simulink model "fuzzy_controller_7_trimf"  (Simulink 7.2)
settings: Solver=ode45  StartTime=0.0  StopTime=10.0  RelTol=1e-3
values from neighbouring files (symbols this model uses):
  fi_1_a = -0.786    [fuzzy_controller_3_trimf_params.m]    (also in fuzzy_controller_5_gbell_params.m = 0.1768; fuzzy_controller_5_trimf_optimal_params.m; fuzzy_controller_5_trimf_params.m; fuzzy_controller_7_trimf_params.m)
  fi_1_b = -0.786    [fuzzy_controller_3_trimf_params.m]    (also in fuzzy_controller_5_gbell_params.m = 3.278; fuzzy_controller_5_trimf_optimal_params.m; fuzzy_controller_5_trimf_params.m; fuzzy_controller_7_trimf_params.m)
  fi_1_c = 0    [fuzzy_controller_3_trimf_params.m]    (also in fuzzy_controller_5_gbell_params.m = -0.7664; fuzzy_controller_5_trimf_optimal_params.m = -0.1; fuzzy_controller_5_trimf_params.m = -0.393; fuzzy_controller_7_trimf_params.m = -0.523)
  fi_2_a = -0.786    [fuzzy_controller_3_trimf_params.m]    (also in fuzzy_controller_5_gbell_params.m = 0.1965; fuzzy_controller_5_trimf_optimal_params.m = -0.1; fuzzy_controller_5_trimf_params.m; fuzzy_controller_7_trimf_params.m)
  fi_2_b = 0    [fuzzy_controller_3_trimf_params.m]    (also in fuzzy_controller_5_gbell_params.m = 3.278; fuzzy_controller_5_trimf_optimal_params.m = -0.05; fuzzy_controller_5_trimf_params.m = -0.393; fuzzy_controller_7_trimf_params.m = -0.5238)
  fi_2_c = 0.786    [fuzzy_controller_3_trimf_params.m]    (also in fuzzy_controller_5_gbell_params.m = -0.393; fuzzy_controller_5_trimf_optimal_params.m = 0; fuzzy_controller_5_trimf_params.m = 0; fuzzy_controller_7_trimf_params.m = -0.262)
  fi_3_a = 0    [fuzzy_controller_3_trimf_params.m]    (also in fuzzy_controller_5_gbell_params.m = 0.1965; fuzzy_controller_5_trimf_optimal_params.m = -0.05; fuzzy_controller_5_trimf_params.m = -0.393; fuzzy_controller_7_trimf_params.m = -0.523)
  fi_3_b = 0.786    [fuzzy_controller_3_trimf_params.m]    (also in fuzzy_controller_5_gbell_params.m = 3.278; fuzzy_controller_5_trimf_optimal_params.m = 0; fuzzy_controller_5_trimf_params.m = 0; fuzzy_controller_7_trimf_params.m = -0.262)
  fi_3_c = 0.786    [fuzzy_controller_3_trimf_params.m]    (also in fuzzy_controller_5_gbell_params.m = 0; fuzzy_controller_5_trimf_optimal_params.m = 0.05; fuzzy_controller_5_trimf_params.m = 0.393; fuzzy_controller_7_trimf_params.m = 0)
  fi_4_a = 0.1965    [fuzzy_controller_5_gbell_params.m]    (also in fuzzy_controller_5_trimf_optimal_params.m = 0; fuzzy_controller_5_trimf_params.m = 0; fuzzy_controller_7_trimf_params.m = -0.262)
  fi_4_b = 3.278    [fuzzy_controller_5_gbell_params.m]    (also in fuzzy_controller_5_trimf_optimal_params.m = 0.05; fuzzy_controller_5_trimf_params.m = 0.393; fuzzy_controller_7_trimf_params.m = 0)
  fi_4_c = 0.393    [fuzzy_controller_5_gbell_params.m]    (also in fuzzy_controller_5_trimf_optimal_params.m = 0.1; fuzzy_controller_5_trimf_params.m = 0.786; fuzzy_controller_7_trimf_params.m = 0.262)
  fi_5_a = 0.1768    [fuzzy_controller_5_gbell_params.m]    (also in fuzzy_controller_5_trimf_optimal_params.m = 0.05; fuzzy_controller_5_trimf_params.m = 0.393; fuzzy_controller_7_trimf_params.m = 0)
  fi_5_b = 3.278    [fuzzy_controller_5_gbell_params.m]    (also in fuzzy_controller_5_trimf_optimal_params.m = 0.1; fuzzy_controller_5_trimf_params.m = 0.786; fuzzy_controller_7_trimf_params.m = 0.262)
  fi_5_c = 0.7664    [fuzzy_controller_5_gbell_params.m]    (also in fuzzy_controller_5_trimf_optimal_params.m = 0.786; fuzzy_controller_5_trimf_params.m = 0.786; fuzzy_controller_7_trimf_params.m = 0.523)
  fi_6_a = 0.262    [fuzzy_controller_7_trimf_params.m]
  fi_6_b = 0.523    [fuzzy_controller_7_trimf_params.m]
  fi_6_c = 0.786    [fuzzy_controller_7_trimf_params.m]
  fi_7_a = 0.523    [fuzzy_controller_7_trimf_params.m]
  fi_7_b = 0.786    [fuzzy_controller_7_trimf_params.m]
  fi_7_c = 0.786    [fuzzy_controller_7_trimf_params.m]
  FORCE_1_a = -150    [fuzzy_controller_3_trimf_params.m]    (also in fuzzy_controller_5_trimf_optimal_params.m; fuzzy_controller_5_trimf_params.m; fuzzy_controller_7_trimf_params.m)
  FORCE_1_b = -150    [fuzzy_controller_3_trimf_params.m]    (also in fuzzy_controller_5_trimf_optimal_params.m; fuzzy_controller_5_trimf_params.m; fuzzy_controller_7_trimf_params.m)
  FORCE_1_c = 0    [fuzzy_controller_3_trimf_params.m]    (also in fuzzy_controller_5_trimf_optimal_params.m = -75; fuzzy_controller_5_trimf_params.m = -75; fuzzy_controller_7_trimf_params.m = -100)
  FORCE_2_a = -150    [fuzzy_controller_3_trimf_params.m]    (also in fuzzy_controller_5_trimf_optimal_params.m; fuzzy_controller_5_trimf_params.m; fuzzy_controller_7_trimf_params.m)
  FORCE_2_b = 0    [fuzzy_controller_3_trimf_params.m]    (also in fuzzy_controller_5_trimf_optimal_params.m = -75; fuzzy_controller_5_trimf_params.m = -75; fuzzy_controller_7_trimf_params.m = -100)
  FORCE_2_c = 150    [fuzzy_controller_3_trimf_params.m]    (also in fuzzy_controller_5_trimf_optimal_params.m = 0; fuzzy_controller_5_trimf_params.m = 0; fuzzy_controller_7_trimf_params.m = -50)
  FORCE_3_a = 0    [fuzzy_controller_3_trimf_params.m]    (also in fuzzy_controller_5_trimf_optimal_params.m = -75; fuzzy_controller_5_trimf_params.m = -75; fuzzy_controller_7_trimf_params.m = -100)
  FORCE_3_b = 150    [fuzzy_controller_3_trimf_params.m]    (also in fuzzy_controller_5_trimf_optimal_params.m = 0; fuzzy_controller_5_trimf_params.m = 0; fuzzy_controller_7_trimf_params.m = -50)
  FORCE_3_c = 150    [fuzzy_controller_3_trimf_params.m]    (also in fuzzy_controller_5_trimf_optimal_params.m = 75; fuzzy_controller_5_trimf_params.m = 75; fuzzy_controller_7_trimf_params.m = 0)
  FORCE_4_a = 0    [fuzzy_controller_5_trimf_optimal_params.m]    (also in fuzzy_controller_5_trimf_params.m; fuzzy_controller_7_trimf_params.m = -50)
  FORCE_4_b = 75    [fuzzy_controller_5_trimf_optimal_params.m]    (also in fuzzy_controller_5_trimf_params.m; fuzzy_controller_7_trimf_params.m = 0)
  FORCE_4_c = 150    [fuzzy_controller_5_trimf_optimal_params.m]    (also in fuzzy_controller_5_trimf_params.m; fuzzy_controller_7_trimf_params.m = 50)
  FORCE_5_a = 75    [fuzzy_controller_5_trimf_optimal_params.m]    (also in fuzzy_controller_5_trimf_params.m; fuzzy_controller_7_trimf_params.m = 0)
  FORCE_5_b = 150    [fuzzy_controller_5_trimf_optimal_params.m]    (also in fuzzy_controller_5_trimf_params.m; fuzzy_controller_7_trimf_params.m = 50)
  FORCE_5_c = 150    [fuzzy_controller_5_trimf_optimal_params.m]    (also in fuzzy_controller_5_trimf_params.m; fuzzy_controller_7_trimf_params.m = 100)
  FORCE_6_a = 50    [fuzzy_controller_7_trimf_params.m]
  FORCE_6_b = 100    [fuzzy_controller_7_trimf_params.m]
  FORCE_6_c = 150    [fuzzy_controller_7_trimf_params.m]
  FORCE_7_a = 100    [fuzzy_controller_7_trimf_params.m]
  FORCE_7_b = 150    [fuzzy_controller_7_trimf_params.m]
  FORCE_7_c = 150    [fuzzy_controller_7_trimf_params.m]
  FORCE_Range_1 = -150    [fuzzy_controller_3_trimf_params.m]    (also in fuzzy_controller_5_gauss_params.m; fuzzy_controller_5_gbell_params.m; fuzzy_controller_5_trimf_optimal_params.m; fuzzy_controller_5_trimf_params.m)
  FORCE_Range_2 = 150    [fuzzy_controller_3_trimf_params.m]    (also in fuzzy_controller_5_gauss_params.m; fuzzy_controller_5_gbell_params.m; fuzzy_controller_5_trimf_optimal_params.m; fuzzy_controller_5_trimf_params.m)
  omega_1_a = -1.57    [fuzzy_controller_3_trimf_params.m]    (also in fuzzy_controller_5_gbell_params.m = 0.3532; fuzzy_controller_5_trimf_optimal_params.m; fuzzy_controller_5_trimf_params.m; fuzzy_controller_7_trimf_params.m)
  omega_1_b = -1.57    [fuzzy_controller_3_trimf_params.m]    (also in fuzzy_controller_5_gbell_params.m = 3.278; fuzzy_controller_5_trimf_optimal_params.m; fuzzy_controller_5_trimf_params.m; fuzzy_controller_7_trimf_params.m)
  omega_1_c = 0    [fuzzy_controller_3_trimf_params.m]    (also in fuzzy_controller_5_gbell_params.m = -1.531; fuzzy_controller_5_trimf_optimal_params.m = -0.86; fuzzy_controller_5_trimf_params.m = -0.785; fuzzy_controller_7_trimf_params.m = -1.047)
  omega_2_a = -1.57    [fuzzy_controller_3_trimf_params.m]    (also in fuzzy_controller_5_gbell_params.m = 0.3925; fuzzy_controller_5_trimf_optimal_params.m = -0.86; fuzzy_controller_5_trimf_params.m; fuzzy_controller_7_trimf_params.m)
  omega_2_b = 0    [fuzzy_controller_3_trimf_params.m]    (also in fuzzy_controller_5_gbell_params.m = 3.278; fuzzy_controller_5_trimf_optimal_params.m = -0.43; fuzzy_controller_5_trimf_params.m = -0.785; fuzzy_controller_7_trimf_params.m = -1.047)
  omega_2_c = 1.57    [fuzzy_controller_3_trimf_params.m]    (also in fuzzy_controller_5_gbell_params.m = -0.785; fuzzy_controller_5_trimf_optimal_params.m = 0; fuzzy_controller_5_trimf_params.m = 0; fuzzy_controller_7_trimf_params.m = -0.523)
  omega_3_a = 0    [fuzzy_controller_3_trimf_params.m]    (also in fuzzy_controller_5_gbell_params.m = 0.3925; fuzzy_controller_5_trimf_optimal_params.m = -0.43; fuzzy_controller_5_trimf_params.m = -0.785; fuzzy_controller_7_trimf_params.m = -1.047)
  omega_3_b = 1.57    [fuzzy_controller_3_trimf_params.m]    (also in fuzzy_controller_5_gbell_params.m = 3.278; fuzzy_controller_5_trimf_optimal_params.m = 0; fuzzy_controller_5_trimf_params.m = 0; fuzzy_controller_7_trimf_params.m = -0.523)
  omega_3_c = 1.57    [fuzzy_controller_3_trimf_params.m]    (also in fuzzy_controller_5_gbell_params.m = 0; fuzzy_controller_5_trimf_optimal_params.m = 0.43; fuzzy_controller_5_trimf_params.m = 0.785; fuzzy_controller_7_trimf_params.m = 0)
  omega_4_a = 0.3925    [fuzzy_controller_5_gbell_params.m]    (also in fuzzy_controller_5_trimf_optimal_params.m = 0; fuzzy_controller_5_trimf_params.m = 0; fuzzy_controller_7_trimf_params.m = -0.523)
  omega_4_b = 3.278    [fuzzy_controller_5_gbell_params.m]    (also in fuzzy_controller_5_trimf_optimal_params.m = 0.43; fuzzy_controller_5_trimf_params.m = 0.785; fuzzy_controller_7_trimf_params.m = 0)
  omega_4_c = 0.785    [fuzzy_controller_5_gbell_params.m]    (also in fuzzy_controller_5_trimf_optimal_params.m = 0.86; fuzzy_controller_5_trimf_params.m = 1.57; fuzzy_controller_7_trimf_params.m = 0.523)
  omega_5_a = 0.3532    [fuzzy_controller_5_gbell_params.m]    (also in fuzzy_controller_5_trimf_optimal_params.m = 0.43; fuzzy_controller_5_trimf_params.m = 0.785; fuzzy_controller_7_trimf_params.m = 0)
  omega_5_b = 3.278    [fuzzy_controller_5_gbell_params.m]    (also in fuzzy_controller_5_trimf_optimal_params.m = 0.86; fuzzy_controller_5_trimf_params.m = 1.57; fuzzy_controller_7_trimf_params.m = 0.523)
  omega_5_c = 1.531    [fuzzy_controller_5_gbell_params.m]    (also in fuzzy_controller_5_trimf_optimal_params.m = 1.57; fuzzy_controller_5_trimf_params.m = 1.57; fuzzy_controller_7_trimf_params.m = 1.047)
  omega_6_a = 0.523    [fuzzy_controller_7_trimf_params.m]
  omega_6_b = 1.047    [fuzzy_controller_7_trimf_params.m]
  omega_6_c = 1.57    [fuzzy_controller_7_trimf_params.m]
  omega_7_a = 1.047    [fuzzy_controller_7_trimf_params.m]
  omega_7_b = 1.57    [fuzzy_controller_7_trimf_params.m]
  omega_7_c = 1.57    [fuzzy_controller_7_trimf_params.m]
(part 1 of 4)
settings Model: Creator=Student  ModifiedByFormat=Student  LastModifiedBy=Student
settings OptimizationCC: ExpressionDepthLimit=128
settings DebuggingCC: AlgebraicLoopMsg=error  UnderspecifiedInitializationDetection=Simplified  MergeDetectMultiDrivingBlocksExec=error  SolverPrmCheckMsg=none  FcnCallInpInsideContextMsg=Enable All  StateNameClashWarn=none  StrictBusMsg=ErrorLevel1
settings HardwareCC: ProdBitPerLong=64  ProdIntDivRoundTo=Zero  ProdEndianess=LittleEndian  ProdWordSize=64  ProdHWDeviceType=Intel->x86-64
settings RTWCC: Description=Create Visual C/C++ Solution File for Simulink Coder  GenerateReport=on  RetainRTWFile=on  LaunchReport=on
settings CodeAppCC: ForceParamTrailComments=on  CustomSymbolStrType=$N$R$M_T
settings GRTTargetCC: TargetFunctionLibrary=C99 (ISO)

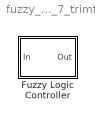
== system fuzzy_controller_7_trimf ==
  Fuzzy Logic Controller : Subsystem

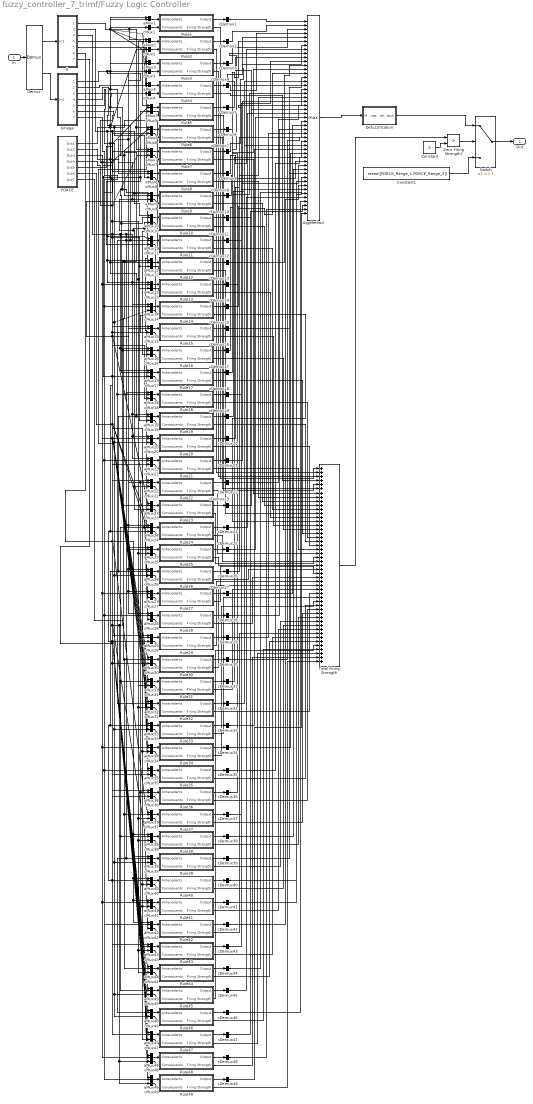
== system fuzzy_controller_7_trimf/Fuzzy Logic Controller ==
  In : Inport
  AggMethod : MinMax  Function=max  Inputs=49  SaturateOnIntegerOverflow=on  InputSameDT=on
  Constant : Constant  Value=0
  Constant1 : Constant  Value=mean([FORCE_Range_1 FORCE_Range_2])
  Defuzzification : Subsystem
  Demux : Demux  Outputs=2
  FORCE : Subsystem
  Rule1 : Subsystem
  Rule10 : Subsystem
  Rule11 : Subsystem
  Rule12 : Subsystem
  Rule13 : Subsystem
  Rule14 : Subsystem
  Rule15 : Subsystem
  Rule16 : Subsystem
  Rule17 : Subsystem
  Rule18 : Subsystem
  Rule19 : Subsystem
  Rule2 : Subsystem
  Rule20 : Subsystem
  Rule21 : Subsystem
  Rule22 : Subsystem
  Rule23 : Subsystem
  Rule24 : Subsystem
  Rule25 : Subsystem
  Rule26 : Subsystem
  Rule27 : Subsystem
  Rule28 : Subsystem
  Rule29 : Subsystem
  Rule3 : Subsystem
  Rule30 : Subsystem
  Rule31 : Subsystem
  Rule32 : Subsystem
  Rule33 : Subsystem
  Rule34 : Subsystem
  Rule35 : Subsystem
  Rule36 : Subsystem
  Rule37 : Subsystem
  Rule38 : Subsystem
  Rule39 : Subsystem
  Rule4 : Subsystem
  Rule40 : Subsystem
  Rule41 : Subsystem
  Rule42 : Subsystem
  Rule43 : Subsystem
  Rule44 : Subsystem
  Rule45 : Subsystem
  Rule46 : Subsystem
  Rule47 : Subsystem
  Rule48 : Subsystem
  Rule49 : Subsystem
  Rule5 : Subsystem
  Rule6 : Subsystem
  Rule7 : Subsystem
  Rule8 : Subsystem
  Rule9 : Subsystem
  Switch : Switch  Threshold=1
  Total Firing Strength : Sum  Inputs=49
  Zero Firing Strength? : RelationalOperator  Operator=>  LogicOutDataTypeMode=boolean  OutDataTypeStr=boolean
  aMux{1..49} (49 alike) : Mux  Inputs=2
  cDemux{1..49} (49 alike) : Demux  Outputs=1
  cMux{1..49} (49 alike) : Mux  Inputs=1
  fi : Subsystem
  omega : Subsystem
  Out : Outport
  wires:
  Total Firing Strength/1 -> Zero Firing Strength?/1
  Constant/1 -> Zero Firing Strength?/2
  Zero Firing Strength?/1 -> Switch/2
  Switch/1 -> Out/1
  Constant1/1 -> Switch/3
  AggMethod/1 -> Defuzzification/1(MF values)
  Defuzzification/1(defuzzified output) -> Switch/1
  Demux/1 -> fi/1(In1)
  In/1 -> Demux/1
  Demux/2 -> omega/1(In1)
  aMux1/1 -> Rule1/1(Antecedents)
  cMux1/1 -> Rule1/2(Consequents)
  fi/1(Out1) -> aMux6/1, aMux7/1, aMux2/1, aMux1/1, aMux3/1, aMux4/1, aMux5/1
  omega/1(Out1) -> aMux36/2, aMux43/2, aMux29/2, aMux22/2, aMux8/2, aMux15/2, aMux1/2
  FORCE/1(Out1) -> cMux15/1, cMux8/1, cMux1/1, cMux2/1
  aMux2/1 -> Rule2/1(Antecedents)
  cMux2/1 -> Rule2/2(Consequents)
  omega/2(Out2) -> aMux16/2, aMux23/2, aMux30/2, aMux37/2, aMux44/2, aMux9/2, aMux2/2
  aMux3/1 -> Rule3/1(Antecedents)
  cMux3/1 -> Rule3/2(Consequents)
  omega/3(Out3) -> aMux10/2, aMux17/2, aMux45/2, aMux38/2, aMux31/2, aMux24/2, aMux3/2
  FORCE/2(Out2) -> cMux22/1, cMux23/1, cMux10/1, cMux16/1, cMux9/1, cMux3/1
  aMux4/1 -> Rule4/1(Antecedents)
  cMux4/1 -> Rule4/2(Consequents)
  omega/4(Out4) -> aMux18/2, aMux25/2, aMux32/2, aMux46/2, aMux39/2, aMux11/2, aMux4/2
  FORCE/3(Out3) -> cMux5/1, cMux11/1, cMux4/1, cMux24/1, cMux30/1, cMux36/1, cMux29/1, cMux17/1
  aMux5/1 -> Rule5/1(Antecedents)
  cMux5/1 -> Rule5/2(Consequents)
  omega/5(Out5) -> aMux5/2, aMux12/2, aMux33/2, aMux47/2, aMux40/2, aMux26/2, aMux19/2
  aMux6/1 -> Rule6/1(Antecedents)
  cMux6/1 -> Rule6/2(Consequents)
  omega/6(Out6) -> aMux48/2, aMux41/2, aMux34/2, aMux27/2, aMux13/2, aMux6/2, aMux20/2
  FORCE/4(Out4) -> cMux19/1, cMux43/1, cMux44/1, cMux38/1, cMux37/1, cMux32/1, cMux25/1, cMux31/1, cMux18/1, cMux12/1, cMux13/1, cMux6/1, cMux7/1
  aMux7/1 -> Rule7/1(Antecedents)
  cMux7/1 -> Rule7/2(Consequents)
  omega/7(Out7) -> aMux49/2, aMux35/2, aMux28/2, aMux21/2, aMux14/2, aMux7/2, aMux42/2
  aMux8/1 -> Rule8/1(Antecedents)
  cMux8/1 -> Rule8/2(Consequents)
  fi/2(Out2) -> aMux9/1, aMux10/1, aMux8/1, aMux13/1, aMux14/1, aMux12/1, aMux11/1
  aMux9/1 -> Rule9/1(Antecedents)
  cMux9/1 -> Rule9/2(Consequents)
  aMux10/1 -> Rule10/1(Antecedents)
  cMux10/1 -> Rule10/2(Consequents)
  aMux11/1 -> Rule11/1(Antecedents)
  cMux11/1 -> Rule11/2(Consequents)
  aMux12/1 -> Rule12/1(Antecedents)
  cMux12/1 -> Rule12/2(Consequents)
  aMux13/1 -> Rule13/1(Antecedents)
  cMux13/1 -> Rule13/2(Consequents)
  aMux14/1 -> Rule14/1(Antecedents)
  cMux14/1 -> Rule14/2(Consequents)
  FORCE/5(Out5) -> cMux26/1, cMux45/1, cMux46/1, cMux39/1, cMux33/1, cMux20/1, cMux14/1
  aMux15/1 -> Rule15/1(Antecedents)
  cMux15/1 -> Rule15/2(Consequents)
  fi/3(Out3) -> aMux21/1, aMux20/1, aMux19/1, aMux18/1, aMux16/1, aMux17/1, aMux15/1
  aMux16/1 -> Rule16/1(Antecedents)
  cMux16/1 -> Rule16/2(Consequents)
  aMux17/1 -> Rule17/1(Antecedents)
  cMux17/1 -> Rule17/2(Consequents)
  aMux18/1 -> Rule18/1(Antecedents)
  cMux18/1 -> Rule18/2(Consequents)
  aMux19/1 -> Rule19/1(Antecedents)
  cMux19/1 -> Rule19/2(Consequents)
  aMux20/1 -> Rule20/1(Antecedents)
  cMux20/1 -> Rule20/2(Consequents)
  aMux21/1 -> Rule21/1(Antecedents)
  cMux21/1 -> Rule21/2(Consequents)
  FORCE/6(Out6) -> cMux41/1, cMux47/1, cMux40/1, cMux34/1, cMux21/1, cMux27/1, cMux28/1
  aMux22/1 -> Rule22/1(Antecedents)
  cMux22/1 -> Rule22/2(Consequents)
  fi/4(Out4) -> aMux27/1, aMux28/1, aMux26/1, aMux25/1, aMux24/1, aMux22/1, aMux23/1
  aMux23/1 -> Rule23/1(Antecedents)
  cMux23/1 -> Rule23/2(Consequents)
  aMux24/1 -> Rule24/1(Antecedents)
  cMux24/1 -> Rule24/2(Consequents)
  aMux25/1 -> Rule25/1(Antecedents)
  cMux25/1 -> Rule25/2(Consequents)
  aMux26/1 -> Rule26/1(Antecedents)
  cMux26/1 -> Rule26/2(Consequents)
  aMux27/1 -> Rule27/1(Antecedents)
  cMux27/1 -> Rule27/2(Consequents)
  aMux28/1 -> Rule28/1(Antecedents)
  cMux28/1 -> Rule28/2(Consequents)
  aMux29/1 -> Rule29/1(Antecedents)
  cMux29/1 -> Rule29/2(Consequents)
  fi/5(Out5) -> aMux29/1, aMux30/1, aMux31/1, aMux32/1, aMux33/1, aMux34/1, aMux35/1
  aMux30/1 -> Rule30/1(Antecedents)
  cMux30/1 -> Rule30/2(Consequents)
  aMux31/1 -> Rule31/1(Antecedents)
  cMux31/1 -> Rule31/2(Consequents)
  aMux32/1 -> Rule32/1(Antecedents)
  cMux32/1 -> Rule32/2(Consequents)
  aMux33/1 -> Rule33/1(Antecedents)
  cMux33/1 -> Rule33/2(Consequents)
  aMux34/1 -> Rule34/1(Antecedents)
  cMux34/1 -> Rule34/2(Consequents)
  aMux35/1 -> Rule35/1(Antecedents)
  cMux35/1 -> Rule35/2(Consequents)
  FORCE/7(Out7) -> cMux48/1, cMux49/1, cMux35/1, cMux42/1
  aMux36/1 -> Rule36/1(Antecedents)
  cMux36/1 -> Rule36/2(Consequents)
  fi/6(Out6) -> aMux38/1, aMux39/1, aMux40/1, aMux41/1, aMux42/1, aMux36/1, aMux37/1
  aMux37/1 -> Rule37/1(Antecedents)
  cMux37/1 -> Rule37/2(Consequents)
  aMux38/1 -> Rule38/1(Antecedents)
  cMux38/1 -> Rule38/2(Consequents)
  aMux39/1 -> Rule39/1(Antecedents)
  cMux39/1 -> Rule39/2(Consequents)
  aMux40/1 -> Rule40/1(Antecedents)
  cMux40/1 -> Rule40/2(Consequents)
  aMux41/1 -> Rule41/1(Antecedents)
  cMux41/1 -> Rule41/2(Consequents)
  aMux42/1 -> Rule42/1(Antecedents)
  cMux42/1 -> Rule42/2(Consequents)
  aMux43/1 -> Rule43/1(Antecedents)
  cMux43/1 -> Rule43/2(Consequents)
  fi/7(Out7) -> aMux43/1, aMux44/1, aMux45/1, aMux46/1, aMux47/1, aMux48/1, aMux49/1
  aMux44/1 -> Rule44/1(Antecedents)
  cMux44/1 -> Rule44/2(Consequents)
  aMux45/1 -> Rule45/1(Antecedents)
  cMux45/1 -> Rule45/2(Consequents)
  aMux46/1 -> Rule46/1(Antecedents)
  cMux46/1 -> Rule46/2(Consequents)
  aMux47/1 -> Rule47/1(Antecedents)
  cMux47/1 -> Rule47/2(Consequents)
  aMux48/1 -> Rule48/1(Antecedents)
  cMux48/1 -> Rule48/2(Consequents)
  aMux49/1 -> Rule49/1(Antecedents)
  cMux49/1 -> Rule49/2(Consequents)
  cDemux1/1 -> AggMethod/1
  cDemux2/1 -> AggMethod/2
  cDemux3/1 -> AggMethod/3
  cDemux4/1 -> AggMethod/4
  cDemux5/1 -> AggMethod/5
  cDemux6/1 -> AggMethod/6
  cDemux7/1 -> AggMethod/7
  cDemux8/1 -> AggMethod/8
  cDemux9/1 -> AggMethod/9
  cDemux10/1 -> AggMethod/10
  cDemux11/1 -> AggMethod/11
  cDemux12/1 -> AggMethod/12
  cDemux13/1 -> AggMethod/13
  cDemux14/1 -> AggMethod/14
  cDemux15/1 -> AggMethod/15
  cDemux16/1 -> AggMethod/16
  cDemux17/1 -> AggMethod/17
  cDemux18/1 -> AggMethod/18
  cDemux19/1 -> AggMethod/19
  cDemux20/1 -> AggMethod/20
  cDemux21/1 -> AggMethod/21
  cDemux22/1 -> AggMethod/22
  cDemux23/1 -> AggMethod/23
  cDemux24/1 -> AggMethod/24
  cDemux25/1 -> AggMethod/25
  cDemux26/1 -> AggMethod/26
  cDemux27/1 -> AggMethod/27
  cDemux28/1 -> AggMethod/28
  cDemux29/1 -> AggMethod/29
  cDemux30/1 -> AggMethod/30
  cDemux31/1 -> AggMethod/31
  cDemux32/1 -> AggMethod/32
  cDemux33/1 -> AggMethod/33
  cDemux34/1 -> AggMethod/34
  cDemux35/1 -> AggMethod/35
  cDemux36/1 -> AggMethod/36
  cDemux37/1 -> AggMethod/37
  cDemux38/1 -> AggMethod/38
  cDemux39/1 -> AggMethod/39
  cDemux40/1 -> AggMethod/40
  cDemux41/1 -> AggMethod/41
  cDemux42/1 -> AggMethod/42
  cDemux43/1 -> AggMethod/43
  cDemux44/1 -> AggMethod/44
  cDemux45/1 -> AggMethod/45
  cDemux46/1 -> AggMethod/46
  cDemux47/1 -> AggMethod/47
  cDemux48/1 -> AggMethod/48
  cDemux49/1 -> AggMethod/49
  Rule1/1(Output) -> cDemux1/1
  Rule2/1(Output) -> cDemux2/1
  Rule3/1(Output) -> cDemux3/1
  Rule4/1(Output) -> cDemux4/1
  Rule5/1(Output) -> cDemux5/1
  Rule6/1(Output) -> cDemux6/1
  Rule49/1(Output) -> cDemux49/1
  Rule48/1(Output) -> cDemux48/1
  Rule47/1(Output) -> cDemux47/1
  Rule46/1(Output) -> cDemux46/1
  Rule45/1(Output) -> cDemux45/1
  Rule44/1(Output) -> cDemux44/1
  Rule42/1(Output) -> cDemux42/1
  Rule41/1(Output) -> cDemux41/1
  Rule43/1(Output) -> cDemux43/1
  Rule40/1(Output) -> cDemux40/1
  Rule39/1(Output) -> cDemux39/1
  Rule38/1(Output) -> cDemux38/1
  Rule36/1(Output) -> cDemux36/1
  Rule37/1(Output) -> cDemux37/1
  Rule35/1(Output) -> cDemux35/1
  Rule34/1(Output) -> cDemux34/1
  Rule33/1(Output) -> cDemux33/1
  Rule31/1(Output) -> cDemux31/1
  Rule32/1(Output) -> cDemux32/1
  Rule30/1(Output) -> cDemux30/1
  Rule29/1(Output) -> cDemux29/1
  Rule28/1(Output) -> cDemux28/1
  Rule27/1(Output) -> cDemux27/1
  Rule26/1(Output) -> cDemux26/1
  Rule25/1(Output) -> cDemux25/1
  Rule24/1(Output) -> cDemux24/1
  Rule23/1(Output) -> cDemux23/1
  Rule22/1(Output) -> cDemux22/1
  Rule21/1(Output) -> cDemux21/1
  Rule20/1(Output) -> cDemux20/1
  Rule19/1(Output) -> cDemux19/1
  Rule18/1(Output) -> cDemux18/1
  Rule17/1(Output) -> cDemux17/1
  Rule16/1(Output) -> cDemux16/1
  Rule15/1(Output) -> cDemux15/1
  Rule14/1(Output) -> cDemux14/1
  Rule13/1(Output) -> cDemux13/1
  Rule7/1(Output) -> cDemux7/1
  Rule8/1(Output) -> cDemux8/1
  Rule9/1(Output) -> cDemux9/1
  Rule10/1(Output) -> cDemux10/1
  Rule11/1(Output) -> cDemux11/1
  Rule12/1(Output) -> cDemux12/1
  Rule1/2(Firing Strength) -> Total Firing Strength/1
  Rule2/2(Firing Strength) -> Total Firing Strength/2
  Rule3/2(Firing Strength) -> Total Firing Strength/3
  Rule4/2(Firing Strength) -> Total Firing Strength/4
  Rule5/2(Firing Strength) -> Total Firing Strength/5
  Rule6/2(Firing Strength) -> Total Firing Strength/6
  Rule7/2(Firing Strength) -> Total Firing Strength/7
  Rule8/2(Firing Strength) -> Total Firing Strength/8
  Rule9/2(Firing Strength) -> Total Firing Strength/9
  Rule10/2(Firing Strength) -> Total Firing Strength/10
  Rule11/2(Firing Strength) -> Total Firing Strength/11
  Rule12/2(Firing Strength) -> Total Firing Strength/12
  Rule13/2(Firing Strength) -> Total Firing Strength/13
  Rule14/2(Firing Strength) -> Total Firing Strength/14
  Rule15/2(Firing Strength) -> Total Firing Strength/15
  Rule16/2(Firing Strength) -> Total Firing Strength/16
  Rule17/2(Firing Strength) -> Total Firing Strength/17
  Rule18/2(Firing Strength) -> Total Firing Strength/18
  Rule19/2(Firing Strength) -> Total Firing Strength/19
  Rule20/2(Firing Strength) -> Total Firing Strength/20
  Rule21/2(Firing Strength) -> Total Firing Strength/21
  Rule22/2(Firing Strength) -> Total Firing Strength/22
  Rule23/2(Firing Strength) -> Total Firing Strength/23
  Rule24/2(Firing Strength) -> Total Firing Strength/24
  Rule25/2(Firing Strength) -> Total Firing Strength/25
  Rule26/2(Firing Strength) -> Total Firing Strength/26
  Rule27/2(Firing Strength) -> Total Firing Strength/27
  Rule28/2(Firing Strength) -> Total Firing Strength/28
  Rule29/2(Firing Strength) -> Total Firing Strength/29
  Rule30/2(Firing Strength) -> Total Firing Strength/30
  Rule31/2(Firing Strength) -> Total Firing Strength/31
  Rule32/2(Firing Strength) -> Total Firing Strength/32
  Rule33/2(Firing Strength) -> Total Firing Strength/33
  Rule34/2(Firing Strength) -> Total Firing Strength/34
  Rule35/2(Firing Strength) -> Total Firing Strength/35
  Rule36/2(Firing Strength) -> Total Firing Strength/36
  Rule37/2(Firing Strength) -> Total Firing Strength/37
  Rule38/2(Firing Strength) -> Total Firing Strength/38
  Rule39/2(Firing Strength) -> Total Firing Strength/39
  Rule40/2(Firing Strength) -> Total Firing Strength/40
  Rule41/2(Firing Strength) -> Total Firing Strength/41
  Rule42/2(Firing Strength) -> Total Firing Strength/42
  Rule43/2(Firing Strength) -> Total Firing Strength/43
  Rule44/2(Firing Strength) -> Total Firing Strength/44
  Rule45/2(Firing Strength) -> Total Firing Strength/45
  Rule46/2(Firing Strength) -> Total Firing Strength/46
  Rule47/2(Firing Strength) -> Total Firing Strength/47
  Rule48/2(Firing Strength) -> Total Firing Strength/48
  Rule49/2(Firing Strength) -> Total Firing Strength/49

== system fuzzy_controller_7_trimf/Fuzzy Logic Controller/Defuzzification ==
  MF values : Inport
  Action: One : Subsystem  TreatAsAtomicUnit=on
  Action: u1 : Subsystem  TreatAsAtomicUnit=on
  Averaging (COA) : Product  Inputs=*/  SaturateOnIntegerOverflow=on  RndMeth=Zero  InputSameDT=on  OutDataTypeStr=Inherit: Same as first input
  Constant1 : Constant  Value=linspace(FORCE_Range_1,FORCE_Range_2,200)
  If : If  IfExpression=u1 <= 0
  Merge : Merge  InitialOutput=0
  Product (COA) : Product  SaturateOnIntegerOverflow=on  RndMeth=Zero  InputSameDT=on  OutDataTypeStr=Inherit: Same as first input
  Sum : Sum  Inputs=+  SaturateOnIntegerOverflow=on  InputSameDT=on  OutDataTypeStr=Inherit: Same as first input
  Sum1 : Sum  Inputs=+  SaturateOnIntegerOverflow=on  InputSameDT=on  OutDataTypeStr=Inherit: Same as first input
  defuzzified output : Outport
  wires:
  Merge/1 -> Averaging (COA)/2
  Action: u1/1(u2) -> Merge/2
  Action: One/1(Out1) -> Merge/1
  If/1 -> Action: One/Action
  If/2 -> Action: u1/Action
  Sum1/1 -> Action: u1/1(u1), If/1
  Constant1/1 -> Product (COA)/1
  Product (COA)/1 -> Sum/1
  MF values/1 -> Product (COA)/2, Sum1/1
  Sum/1 -> Averaging (COA)/1
  Averaging (COA)/1 -> defuzzified output/1

== system fuzzy_controller_7_trimf/Fuzzy Logic Controller/FORCE ==
  Constant2 : Constant  Value=linspace(FORCE_Range_1,FORCE_Range_2,200)
  tri mf1 : Subsystem  mask{a=FORCE_1_a, b=FORCE_1_b, c=FORCE_1_c}
      mask prompts: a "Left base point a:"; b "Peak location b:"; c "Right base point c:"
  tri mf2 : Subsystem  mask{a=FORCE_2_a, b=FORCE_2_b, c=FORCE_2_c}
      mask prompts: a "Left base point a:"; b "Peak location b:"; c "Right base point c:"
  tri mf3 : Subsystem  mask{a=FORCE_3_a, b=FORCE_3_b, c=FORCE_3_c}
      mask prompts: a "Left base point a:"; b "Peak location b:"; c "Right base point c:"
  tri mf4 : Subsystem  mask{a=FORCE_4_a, b=FORCE_4_b, c=FORCE_4_c}
      mask prompts: a "Left base point a:"; b "Peak location b:"; c "Right base point c:"
  tri mf5 : Subsystem  mask{a=FORCE_5_a, b=FORCE_5_b, c=FORCE_5_c}
      mask prompts: a "Left base point a:"; b "Peak location b:"; c "Right base point c:"
  tri mf6 : Subsystem  mask{a=FORCE_6_a, b=FORCE_6_b, c=FORCE_6_c}
      mask prompts: a "Left base point a:"; b "Peak location b:"; c "Right base point c:"
  tri mf7 : Subsystem  mask{a=FORCE_7_a, b=FORCE_7_b, c=FORCE_7_c}
      mask prompts: a "Left base point a:"; b "Peak location b:"; c "Right base point c:"
  Out1 : Outport
  Out2 : Outport  Port=2
  Out3 : Outport  Port=3
  Out4 : Outport  Port=4
  Out5 : Outport  Port=5
  Out6 : Outport  Port=6
  Out7 : Outport  Port=7
  wires:
  Constant2/1 -> tri mf4/1(x), tri mf6/1(x), tri mf7/1(x), tri mf5/1(x), tri mf3/1(x), tri mf1/1(x), tri mf2/1(x)
  tri mf1/1(MF) -> Out1/1
  tri mf2/1(MF) -> Out2/1
  tri mf3/1(MF) -> Out3/1
  tri mf4/1(MF) -> Out4/1
  tri mf5/1(MF) -> Out5/1
  tri mf6/1(MF) -> Out6/1
  tri mf7/1(MF) -> Out7/1

== system fuzzy_controller_7_trimf/Fuzzy Logic Controller/Rule1 ==
  Antecedents : Inport
  Consequents : Inport  Port=2
  Weight : Constant
  Weighting : Product  SaturateOnIntegerOverflow=on  RndMeth=Zero  InputSameDT=on  OutDataTypeStr=Inherit: Same as first input
  andorMethod : MinMax  SaturateOnIntegerOverflow=on  InputSameDT=on
  impMethod : MinMax  Inputs=2  SaturateOnIntegerOverflow=on  InputSameDT=on
  Output : Outport
  Firing Strength : Outport  Port=2
  wires:
  impMethod/1 -> Output/1
  Weighting/1 -> Firing Strength/1, impMethod/1
  Consequents/1 -> impMethod/2
  Weight/1 -> Weighting/1
  andorMethod/1 -> Weighting/2
  Antecedents/1 -> andorMethod/1

== system fuzzy_controller_7_trimf/Fuzzy Logic Controller/Rule10 ==
  Antecedents : Inport
  Consequents : Inport  Port=2
  Weight : Constant
  Weighting : Product  SaturateOnIntegerOverflow=on  RndMeth=Zero  InputSameDT=on  OutDataTypeStr=Inherit: Same as first input
  andorMethod : MinMax  SaturateOnIntegerOverflow=on  InputSameDT=on
  impMethod : MinMax  Inputs=2  SaturateOnIntegerOverflow=on  InputSameDT=on
  Output : Outport
  Firing Strength : Outport  Port=2
  wires:
  impMethod/1 -> Output/1
  Weighting/1 -> Firing Strength/1, impMethod/1
  Consequents/1 -> impMethod/2
  Weight/1 -> Weighting/1
  andorMethod/1 -> Weighting/2
  Antecedents/1 -> andorMethod/1

== system fuzzy_controller_7_trimf/Fuzzy Logic Controller/Rule11 ==
  Antecedents : Inport
  Consequents : Inport  Port=2
  Weight : Constant
  Weighting : Product  SaturateOnIntegerOverflow=on  RndMeth=Zero  InputSameDT=on  OutDataTypeStr=Inherit: Same as first input
  andorMethod : MinMax  SaturateOnIntegerOverflow=on  InputSameDT=on
  impMethod : MinMax  Inputs=2  SaturateOnIntegerOverflow=on  InputSameDT=on
  Output : Outport
  Firing Strength : Outport  Port=2
  wires:
  impMethod/1 -> Output/1
  Weighting/1 -> Firing Strength/1, impMethod/1
  Consequents/1 -> impMethod/2
  Weight/1 -> Weighting/1
  andorMethod/1 -> Weighting/2
  Antecedents/1 -> andorMethod/1

== system fuzzy_controller_7_trimf/Fuzzy Logic Controller/Rule12 ==
  Antecedents : Inport
  Consequents : Inport  Port=2
  Weight : Constant
  Weighting : Product  SaturateOnIntegerOverflow=on  RndMeth=Zero  InputSameDT=on  OutDataTypeStr=Inherit: Same as first input
  andorMethod : MinMax  SaturateOnIntegerOverflow=on  InputSameDT=on
  impMethod : MinMax  Inputs=2  SaturateOnIntegerOverflow=on  InputSameDT=on
  Output : Outport
  Firing Strength : Outport  Port=2
  wires:
  impMethod/1 -> Output/1
  Weighting/1 -> Firing Strength/1, impMethod/1
  Consequents/1 -> impMethod/2
  Weight/1 -> Weighting/1
  andorMethod/1 -> Weighting/2
  Antecedents/1 -> andorMethod/1

== system fuzzy_controller_7_trimf/Fuzzy Logic Controller/Rule13 ==
  Antecedents : Inport
  Consequents : Inport  Port=2
  Weight : Constant
  Weighting : Product  SaturateOnIntegerOverflow=on  RndMeth=Zero  InputSameDT=on  OutDataTypeStr=Inherit: Same as first input
  andorMethod : MinMax  SaturateOnIntegerOverflow=on  InputSameDT=on
  impMethod : MinMax  Inputs=2  SaturateOnIntegerOverflow=on  InputSameDT=on
  Output : Outport
  Firing Strength : Outport  Port=2
  wires:
  impMethod/1 -> Output/1
  Weighting/1 -> Firing Strength/1, impMethod/1
  Consequents/1 -> impMethod/2
  Weight/1 -> Weighting/1
  andorMethod/1 -> Weighting/2
  Antecedents/1 -> andorMethod/1

== system fuzzy_controller_7_trimf/Fuzzy Logic Controller/Rule14 ==
  Antecedents : Inport
  Consequents : Inport  Port=2
  Weight : Constant
  Weighting : Product  SaturateOnIntegerOverflow=on  RndMeth=Zero  InputSameDT=on  OutDataTypeStr=Inherit: Same as first input
  andorMethod : MinMax  SaturateOnIntegerOverflow=on  InputSameDT=on
  impMethod : MinMax  Inputs=2  SaturateOnIntegerOverflow=on  InputSameDT=on
  Output : Outport
  Firing Strength : Outport  Port=2
  wires:
  impMethod/1 -> Output/1
  Weighting/1 -> Firing Strength/1, impMethod/1
  Consequents/1 -> impMethod/2
  Weight/1 -> Weighting/1
  andorMethod/1 -> Weighting/2
  Antecedents/1 -> andorMethod/1

== system fuzzy_controller_7_trimf/Fuzzy Logic Controller/Rule15 ==
  Antecedents : Inport
  Consequents : Inport  Port=2
  Weight : Constant
  Weighting : Product  SaturateOnIntegerOverflow=on  RndMeth=Zero  InputSameDT=on  OutDataTypeStr=Inherit: Same as first input
  andorMethod : MinMax  SaturateOnIntegerOverflow=on  InputSameDT=on
  impMethod : MinMax  Inputs=2  SaturateOnIntegerOverflow=on  InputSameDT=on
  Output : Outport
  Firing Strength : Outport  Port=2
  wires:
  impMethod/1 -> Output/1
  Weighting/1 -> Firing Strength/1, impMethod/1
  Consequents/1 -> impMethod/2
  Weight/1 -> Weighting/1
  andorMethod/1 -> Weighting/2
  Antecedents/1 -> andorMethod/1

== system fuzzy_controller_7_trimf/Fuzzy Logic Controller/Rule16 ==
  Antecedents : Inport
  Consequents : Inport  Port=2
  Weight : Constant
  Weighting : Product  SaturateOnIntegerOverflow=on  RndMeth=Zero  InputSameDT=on  OutDataTypeStr=Inherit: Same as first input
  andorMethod : MinMax  SaturateOnIntegerOverflow=on  InputSameDT=on
  impMethod : MinMax  Inputs=2  SaturateOnIntegerOverflow=on  InputSameDT=on
  Output : Outport
  Firing Strength : Outport  Port=2
  wires:
  impMethod/1 -> Output/1
  Weighting/1 -> Firing Strength/1, impMethod/1
  Consequents/1 -> impMethod/2
  Weight/1 -> Weighting/1
  andorMethod/1 -> Weighting/2
  Antecedents/1 -> andorMethod/1

== system fuzzy_controller_7_trimf/Fuzzy Logic Controller/Rule17 ==
  Antecedents : Inport
  Consequents : Inport  Port=2
  Weight : Constant
  Weighting : Product  SaturateOnIntegerOverflow=on  RndMeth=Zero  InputSameDT=on  OutDataTypeStr=Inherit: Same as first input
  andorMethod : MinMax  SaturateOnIntegerOverflow=on  InputSameDT=on
  impMethod : MinMax  Inputs=2  SaturateOnIntegerOverflow=on  InputSameDT=on
  Output : Outport
  Firing Strength : Outport  Port=2
  wires:
  impMethod/1 -> Output/1
  Weighting/1 -> Firing Strength/1, impMethod/1
  Consequents/1 -> impMethod/2
  Weight/1 -> Weighting/1
  andorMethod/1 -> Weighting/2
  Antecedents/1 -> andorMethod/1

== system fuzzy_controller_7_trimf/Fuzzy Logic Controller/Rule18 ==
  Antecedents : Inport
  Consequents : Inport  Port=2
  Weight : Constant
  Weighting : Product  SaturateOnIntegerOverflow=on  RndMeth=Zero  InputSameDT=on  OutDataTypeStr=Inherit: Same as first input
  andorMethod : MinMax  SaturateOnIntegerOverflow=on  InputSameDT=on
  impMethod : MinMax  Inputs=2  SaturateOnIntegerOverflow=on  InputSameDT=on
  Output : Outport
  Firing Strength : Outport  Port=2
  wires:
  impMethod/1 -> Output/1
  Weighting/1 -> Firing Strength/1, impMethod/1
  Consequents/1 -> impMethod/2
  Weight/1 -> Weighting/1
  andorMethod/1 -> Weighting/2
  Antecedents/1 -> andorMethod/1

== system fuzzy_controller_7_trimf/Fuzzy Logic Controller/Rule19 ==
  Antecedents : Inport
  Consequents : Inport  Port=2
  Weight : Constant
  Weighting : Product  SaturateOnIntegerOverflow=on  RndMeth=Zero  InputSameDT=on  OutDataTypeStr=Inherit: Same as first input
  andorMethod : MinMax  SaturateOnIntegerOverflow=on  InputSameDT=on
  impMethod : MinMax  Inputs=2  SaturateOnIntegerOverflow=on  InputSameDT=on
  Output : Outport
  Firing Strength : Outport  Port=2
  wires:
  impMethod/1 -> Output/1
  Weighting/1 -> Firing Strength/1, impMethod/1
  Consequents/1 -> impMethod/2
  Weight/1 -> Weighting/1
  andorMethod/1 -> Weighting/2
  Antecedents/1 -> andorMethod/1

== system fuzzy_controller_7_trimf/Fuzzy Logic Controller/Rule2 ==
  Antecedents : Inport
  Consequents : Inport  Port=2
  Weight : Constant
  Weighting : Product  SaturateOnIntegerOverflow=on  RndMeth=Zero  InputSameDT=on  OutDataTypeStr=Inherit: Same as first input
  andorMethod : MinMax  SaturateOnIntegerOverflow=on  InputSameDT=on
  impMethod : MinMax  Inputs=2  SaturateOnIntegerOverflow=on  InputSameDT=on
  Output : Outport
  Firing Strength : Outport  Port=2
  wires:
  impMethod/1 -> Output/1
  Weighting/1 -> Firing Strength/1, impMethod/1
  Consequents/1 -> impMethod/2
  Weight/1 -> Weighting/1
  andorMethod/1 -> Weighting/2
  Antecedents/1 -> andorMethod/1

== system fuzzy_controller_7_trimf/Fuzzy Logic Controller/Rule20 ==
  Antecedents : Inport
  Consequents : Inport  Port=2
  Weight : Constant
  Weighting : Product  SaturateOnIntegerOverflow=on  RndMeth=Zero  InputSameDT=on  OutDataTypeStr=Inherit: Same as first input
  andorMethod : MinMax  SaturateOnIntegerOverflow=on  InputSameDT=on
  impMethod : MinMax  Inputs=2  SaturateOnIntegerOverflow=on  InputSameDT=on
  Output : Outport
  Firing Strength : Outport  Port=2
  wires:
  impMethod/1 -> Output/1
  Weighting/1 -> Firing Strength/1, impMethod/1
  Consequents/1 -> impMethod/2
  Weight/1 -> Weighting/1
  andorMethod/1 -> Weighting/2
  Antecedents/1 -> andorMethod/1

== system fuzzy_controller_7_trimf/Fuzzy Logic Controller/Rule21 ==
  Antecedents : Inport
  Consequents : Inport  Port=2
  Weight : Constant
  Weighting : Product  SaturateOnIntegerOverflow=on  RndMeth=Zero  InputSameDT=on  OutDataTypeStr=Inherit: Same as first input
  andorMethod : MinMax  SaturateOnIntegerOverflow=on  InputSameDT=on
  impMethod : MinMax  Inputs=2  SaturateOnIntegerOverflow=on  InputSameDT=on
  Output : Outport
  Firing Strength : Outport  Port=2
  wires:
  impMethod/1 -> Output/1
  Weighting/1 -> Firing Strength/1, impMethod/1
  Consequents/1 -> impMethod/2
  Weight/1 -> Weighting/1
  andorMethod/1 -> Weighting/2
  Antecedents/1 -> andorMethod/1

== system fuzzy_controller_7_trimf/Fuzzy Logic Controller/Rule22 ==
  Antecedents : Inport
  Consequents : Inport  Port=2
  Weight : Constant
  Weighting : Product  SaturateOnIntegerOverflow=on  RndMeth=Zero  InputSameDT=on  OutDataTypeStr=Inherit: Same as first input
  andorMethod : MinMax  SaturateOnIntegerOverflow=on  InputSameDT=on
  impMethod : MinMax  Inputs=2  SaturateOnIntegerOverflow=on  InputSameDT=on
  Output : Outport
  Firing Strength : Outport  Port=2
  wires:
  impMethod/1 -> Output/1
  Weighting/1 -> Firing Strength/1, impMethod/1
  Consequents/1 -> impMethod/2
  Weight/1 -> Weighting/1
  andorMethod/1 -> Weighting/2
  Antecedents/1 -> andorMethod/1

== system fuzzy_controller_7_trimf/Fuzzy Logic Controller/Rule23 ==
  Antecedents : Inport
  Consequents : Inport  Port=2
  Weight : Constant
  Weighting : Product  SaturateOnIntegerOverflow=on  RndMeth=Zero  InputSameDT=on  OutDataTypeStr=Inherit: Same as first input
  andorMethod : MinMax  SaturateOnIntegerOverflow=on  InputSameDT=on
  impMethod : MinMax  Inputs=2  SaturateOnIntegerOverflow=on  InputSameDT=on
  Output : Outport
  Firing Strength : Outport  Port=2
  wires:
  impMethod/1 -> Output/1
  Weighting/1 -> Firing Strength/1, impMethod/1
  Consequents/1 -> impMethod/2
  Weight/1 -> Weighting/1
  andorMethod/1 -> Weighting/2
  Antecedents/1 -> andorMethod/1

== system fuzzy_controller_7_trimf/Fuzzy Logic Controller/Rule24 ==
  Antecedents : Inport
  Consequents : Inport  Port=2
  Weight : Constant
  Weighting : Product  SaturateOnIntegerOverflow=on  RndMeth=Zero  InputSameDT=on  OutDataTypeStr=Inherit: Same as first input
  andorMethod : MinMax  SaturateOnIntegerOverflow=on  InputSameDT=on
  impMethod : MinMax  Inputs=2  SaturateOnIntegerOverflow=on  InputSameDT=on
  Output : Outport
  Firing Strength : Outport  Port=2
  wires:
  impMethod/1 -> Output/1
  Weighting/1 -> Firing Strength/1, impMethod/1
  Consequents/1 -> impMethod/2
  Weight/1 -> Weighting/1
  andorMethod/1 -> Weighting/2
  Antecedents/1 -> andorMethod/1

== system fuzzy_controller_7_trimf/Fuzzy Logic Controller/Rule25 ==
  Antecedents : Inport
  Consequents : Inport  Port=2
  Weight : Constant
  Weighting : Product  SaturateOnIntegerOverflow=on  RndMeth=Zero  InputSameDT=on  OutDataTypeStr=Inherit: Same as first input
  andorMethod : MinMax  SaturateOnIntegerOverflow=on  InputSameDT=on
  impMethod : MinMax  Inputs=2  SaturateOnIntegerOverflow=on  InputSameDT=on
  Output : Outport
  Firing Strength : Outport  Port=2
  wires:
  impMethod/1 -> Output/1
  Weighting/1 -> Firing Strength/1, impMethod/1
  Consequents/1 -> impMethod/2
  Weight/1 -> Weighting/1
  andorMethod/1 -> Weighting/2
  Antecedents/1 -> andorMethod/1

== system fuzzy_controller_7_trimf/Fuzzy Logic Controller/Rule26 ==
  Antecedents : Inport
  Consequents : Inport  Port=2
  Weight : Constant
  Weighting : Product  SaturateOnIntegerOverflow=on  RndMeth=Zero  InputSameDT=on  OutDataTypeStr=Inherit: Same as first input
  andorMethod : MinMax  SaturateOnIntegerOverflow=on  InputSameDT=on
  impMethod : MinMax  Inputs=2  SaturateOnIntegerOverflow=on  InputSameDT=on
  Output : Outport
  Firing Strength : Outport  Port=2
  wires:
  impMethod/1 -> Output/1
  Weighting/1 -> Firing Strength/1, impMethod/1
  Consequents/1 -> impMethod/2
  Weight/1 -> Weighting/1
  andorMethod/1 -> Weighting/2
  Antecedents/1 -> andorMethod/1

== system fuzzy_controller_7_trimf/Fuzzy Logic Controller/Rule27 ==
  Antecedents : Inport
  Consequents : Inport  Port=2
  Weight : Constant
  Weighting : Product  SaturateOnIntegerOverflow=on  RndMeth=Zero  InputSameDT=on  OutDataTypeStr=Inherit: Same as first input
  andorMethod : MinMax  SaturateOnIntegerOverflow=on  InputSameDT=on
  impMethod : MinMax  Inputs=2  SaturateOnIntegerOverflow=on  InputSameDT=on
  Output : Outport
  Firing Strength : Outport  Port=2
  wires:
  impMethod/1 -> Output/1
  Weighting/1 -> Firing Strength/1, impMethod/1
  Consequents/1 -> impMethod/2
  Weight/1 -> Weighting/1
  andorMethod/1 -> Weighting/2
  Antecedents/1 -> andorMethod/1

== system fuzzy_controller_7_trimf/Fuzzy Logic Controller/Rule28 ==
  Antecedents : Inport
  Consequents : Inport  Port=2
  Weight : Constant
  Weighting : Product  SaturateOnIntegerOverflow=on  RndMeth=Zero  InputSameDT=on  OutDataTypeStr=Inherit: Same as first input
  andorMethod : MinMax  SaturateOnIntegerOverflow=on  InputSameDT=on
  impMethod : MinMax  Inputs=2  SaturateOnIntegerOverflow=on  InputSameDT=on
  Output : Outport
  Firing Strength : Outport  Port=2
  wires:
  impMethod/1 -> Output/1
  Weighting/1 -> Firing Strength/1, impMethod/1
  Consequents/1 -> impMethod/2
  Weight/1 -> Weighting/1
  andorMethod/1 -> Weighting/2
  Antecedents/1 -> andorMethod/1

== system fuzzy_controller_7_trimf/Fuzzy Logic Controller/Rule29 ==
  Antecedents : Inport
  Consequents : Inport  Port=2
  Weight : Constant
  Weighting : Product  SaturateOnIntegerOverflow=on  RndMeth=Zero  InputSameDT=on  OutDataTypeStr=Inherit: Same as first input
  andorMethod : MinMax  SaturateOnIntegerOverflow=on  InputSameDT=on
  impMethod : MinMax  Inputs=2  SaturateOnIntegerOverflow=on  InputSameDT=on
  Output : Outport
  Firing Strength : Outport  Port=2
  wires:
  impMethod/1 -> Output/1
  Weighting/1 -> Firing Strength/1, impMethod/1
  Consequents/1 -> impMethod/2
  Weight/1 -> Weighting/1
  andorMethod/1 -> Weighting/2
  Antecedents/1 -> andorMethod/1

== system fuzzy_controller_7_trimf/Fuzzy Logic Controller/Rule3 ==
  Antecedents : Inport
  Consequents : Inport  Port=2
  Weight : Constant
  Weighting : Product  SaturateOnIntegerOverflow=on  RndMeth=Zero  InputSameDT=on  OutDataTypeStr=Inherit: Same as first input
  andorMethod : MinMax  SaturateOnIntegerOverflow=on  InputSameDT=on
  impMethod : MinMax  Inputs=2  SaturateOnIntegerOverflow=on  InputSameDT=on
  Output : Outport
  Firing Strength : Outport  Port=2
  wires:
  impMethod/1 -> Output/1
  Weighting/1 -> Firing Strength/1, impMethod/1
  Consequents/1 -> impMethod/2
  Weight/1 -> Weighting/1
  andorMethod/1 -> Weighting/2
  Antecedents/1 -> andorMethod/1

== system fuzzy_controller_7_trimf/Fuzzy Logic Controller/Rule30 ==
  Antecedents : Inport
  Consequents : Inport  Port=2
  Weight : Constant
  Weighting : Product  SaturateOnIntegerOverflow=on  RndMeth=Zero  InputSameDT=on  OutDataTypeStr=Inherit: Same as first input
  andorMethod : MinMax  SaturateOnIntegerOverflow=on  InputSameDT=on
  impMethod : MinMax  Inputs=2  SaturateOnIntegerOverflow=on  InputSameDT=on
  Output : Outport
  Firing Strength : Outport  Port=2
  wires:
  impMethod/1 -> Output/1
  Weighting/1 -> Firing Strength/1, impMethod/1
  Consequents/1 -> impMethod/2
  Weight/1 -> Weighting/1
  andorMethod/1 -> Weighting/2
  Antecedents/1 -> andorMethod/1

== system fuzzy_controller_7_trimf/Fuzzy Logic Controller/Rule31 ==
  Antecedents : Inport
  Consequents : Inport  Port=2
  Weight : Constant
  Weighting : Product  SaturateOnIntegerOverflow=on  RndMeth=Zero  InputSameDT=on  OutDataTypeStr=Inherit: Same as first input
  andorMethod : MinMax  SaturateOnIntegerOverflow=on  InputSameDT=on
  impMethod : MinMax  Inputs=2  SaturateOnIntegerOverflow=on  InputSameDT=on
  Output : Outport
  Firing Strength : Outport  Port=2
  wires:
  impMethod/1 -> Output/1
  Weighting/1 -> Firing Strength/1, impMethod/1
  Consequents/1 -> impMethod/2
  Weight/1 -> Weighting/1
  andorMethod/1 -> Weighting/2
  Antecedents/1 -> andorMethod/1

== system fuzzy_controller_7_trimf/Fuzzy Logic Controller/Rule32 ==
  Antecedents : Inport
  Consequents : Inport  Port=2
  Weight : Constant
  Weighting : Product  SaturateOnIntegerOverflow=on  RndMeth=Zero  InputSameDT=on  OutDataTypeStr=Inherit: Same as first input
  andorMethod : MinMax  SaturateOnIntegerOverflow=on  InputSameDT=on
  impMethod : MinMax  Inputs=2  SaturateOnIntegerOverflow=on  InputSameDT=on
  Output : Outport
  Firing Strength : Outport  Port=2
  wires:
  impMethod/1 -> Output/1
  Weighting/1 -> Firing Strength/1, impMethod/1
  Consequents/1 -> impMethod/2
  Weight/1 -> Weighting/1
  andorMethod/1 -> Weighting/2
  Antecedents/1 -> andorMethod/1

== system fuzzy_controller_7_trimf/Fuzzy Logic Controller/Rule33 ==
  Antecedents : Inport
  Consequents : Inport  Port=2
  Weight : Constant
  Weighting : Product  SaturateOnIntegerOverflow=on  RndMeth=Zero  InputSameDT=on  OutDataTypeStr=Inherit: Same as first input
  andorMethod : MinMax  SaturateOnIntegerOverflow=on  InputSameDT=on
  impMethod : MinMax  Inputs=2  SaturateOnIntegerOverflow=on  InputSameDT=on
  Output : Outport
  Firing Strength : Outport  Port=2
  wires:
  impMethod/1 -> Output/1
  Weighting/1 -> Firing Strength/1, impMethod/1
  Consequents/1 -> impMethod/2
  Weight/1 -> Weighting/1
  andorMethod/1 -> Weighting/2
  Antecedents/1 -> andorMethod/1

== system fuzzy_controller_7_trimf/Fuzzy Logic Controller/Rule34 ==
  Antecedents : Inport
  Consequents : Inport  Port=2
  Weight : Constant
  Weighting : Product  SaturateOnIntegerOverflow=on  RndMeth=Zero  InputSameDT=on  OutDataTypeStr=Inherit: Same as first input
  andorMethod : MinMax  SaturateOnIntegerOverflow=on  InputSameDT=on
  impMethod : MinMax  Inputs=2  SaturateOnIntegerOverflow=on  InputSameDT=on
  Output : Outport
  Firing Strength : Outport  Port=2
  wires:
  impMethod/1 -> Output/1
  Weighting/1 -> Firing Strength/1, impMethod/1
  Consequents/1 -> impMethod/2
  Weight/1 -> Weighting/1
  andorMethod/1 -> Weighting/2
  Antecedents/1 -> andorMethod/1

== system fuzzy_controller_7_trimf/Fuzzy Logic Controller/Rule35 ==
  Antecedents : Inport
  Consequents : Inport  Port=2
  Weight : Constant
  Weighting : Product  SaturateOnIntegerOverflow=on  RndMeth=Zero  InputSameDT=on  OutDataTypeStr=Inherit: Same as first input
  andorMethod : MinMax  SaturateOnIntegerOverflow=on  InputSameDT=on
  impMethod : MinMax  Inputs=2  SaturateOnIntegerOverflow=on  InputSameDT=on
  Output : Outport
  Firing Strength : Outport  Port=2
  wires:
  impMethod/1 -> Output/1
  Weighting/1 -> Firing Strength/1, impMethod/1
  Consequents/1 -> impMethod/2
  Weight/1 -> Weighting/1
  andorMethod/1 -> Weighting/2
  Antecedents/1 -> andorMethod/1

== system fuzzy_controller_7_trimf/Fuzzy Logic Controller/Rule36 ==
  Antecedents : Inport
  Consequents : Inport  Port=2
  Weight : Constant
  Weighting : Product  SaturateOnIntegerOverflow=on  RndMeth=Zero  InputSameDT=on  OutDataTypeStr=Inherit: Same as first input
  andorMethod : MinMax  SaturateOnIntegerOverflow=on  InputSameDT=on
  impMethod : MinMax  Inputs=2  SaturateOnIntegerOverflow=on  InputSameDT=on
  Output : Outport
  Firing Strength : Outport  Port=2
  wires:
  impMethod/1 -> Output/1
  Weighting/1 -> Firing Strength/1, impMethod/1
  Consequents/1 -> impMethod/2
  Weight/1 -> Weighting/1
  andorMethod/1 -> Weighting/2
  Antecedents/1 -> andorMethod/1

== system fuzzy_controller_7_trimf/Fuzzy Logic Controller/Rule37 ==
  Antecedents : Inport
  Consequents : Inport  Port=2
  Weight : Constant
  Weighting : Product  SaturateOnIntegerOverflow=on  RndMeth=Zero  InputSameDT=on  OutDataTypeStr=Inherit: Same as first input
  andorMethod : MinMax  SaturateOnIntegerOverflow=on  InputSameDT=on
  impMethod : MinMax  Inputs=2  SaturateOnIntegerOverflow=on  InputSameDT=on
  Output : Outport
  Firing Strength : Outport  Port=2
  wires:
  impMethod/1 -> Output/1
  Weighting/1 -> Firing Strength/1, impMethod/1
  Consequents/1 -> impMethod/2
  Weight/1 -> Weighting/1
  andorMethod/1 -> Weighting/2
  Antecedents/1 -> andorMethod/1

== system fuzzy_controller_7_trimf/Fuzzy Logic Controller/Rule38 ==
  Antecedents : Inport
  Consequents : Inport  Port=2
  Weight : Constant
  Weighting : Product  SaturateOnIntegerOverflow=on  RndMeth=Zero  InputSameDT=on  OutDataTypeStr=Inherit: Same as first input
  andorMethod : MinMax  SaturateOnIntegerOverflow=on  InputSameDT=on
  impMethod : MinMax  Inputs=2  SaturateOnIntegerOverflow=on  InputSameDT=on
  Output : Outport
  Firing Strength : Outport  Port=2
  wires:
  impMethod/1 -> Output/1
  Weighting/1 -> Firing Strength/1, impMethod/1
  Consequents/1 -> impMethod/2
  Weight/1 -> Weighting/1
  andorMethod/1 -> Weighting/2
  Antecedents/1 -> andorMethod/1
